simulink model "benchlink"  (R2024b)
settings: Solver=FixedStepDiscrete  StartTime=0.0  StopTime=0.005*16  RelTol=1e-3
model workspace (MAT data in the model file):
  socvcb : containers.Map (value not decoded)
values from neighbouring files (symbols this model uses):
  access = [32 0 4 36 32 0 4 36 32 0 4 36 ... (16 elements, 16x1)]    [all_variables.mat]
  qam_params =     [all_variables.mat]
undefined symbols (not defined in the file or in its folder): Add, j, QAM, rms, Shift
libraries: hdlsllib x53, simulink_need_slupdate x22, simulink x18, dspsigops x16, commdigbbndam3 x6, dsphdlmathfun2 x2, commchan3 x1, commrflib2 x1, dsphdlsigops2 x1, dspstat3 x1, dsphdlfiltering2 x1, simulink_extras x1
(part 3 of 5)

== system benchlink/HDL_64QAM/HDLRxIPCore/QAM Rx HDL/DA CFC_Avg/Moving_Average ==
  dataIn : Inport
  Trigger : TriggerPort  VariantControl=(inherit)  PortDimensions=1
  Add1 : Sum  Inputs=+-+  OutDataTypeStr=uint16
  Constant18 : Constant  Value=0.125  OutDataTypeStr=fixdt(1,16,14)  SampleTime=-1
  Delay : Delay  DelayLength=8
  Delay4 : Delay  DelayLength=1  InitialCondition=0  UseCircularBuffer=on
  Product : Product
  Time Scope : Scope  NumInputPorts=4
  to int1 : DataTypeConversion  OutDataTypeStr=int16  RndMeth=Floor
  to int2 : DataTypeConversion  Commented=through  OutDataTypeStr=int32  RndMeth=Floor
  dataOut : Outport  InitialOutput=0  VectorParamsAs1DForOutWhenUnconnected=off
  wires:
  dataIn/1 -> to int2/1
  Delay4/1 -> Add1/1
  Product/1 -> to int1/1
  to int1/1 -> Time Scope/4, dataOut/1
  Delay/1 -> Time Scope/2, Add1/2
  Add1/1 -> Time Scope/3, Product/1, Delay4/1
  to int2/1 -> Time Scope/1, Add1/3, Delay/1
  Constant18/1 -> Product/2

== system benchlink/HDL_64QAM/HDLRxIPCore/QAM Rx HDL/EB Downsampler by 6/Modulus ==
  note: sqrt(I^2+Q^2) can be approximated as |L|+0.4*|S|,
      | where |L| is the absolute value of the larger of I or Q,
      | and |S| is the absolute value of the smaller of I or Q.
      |
      | See "|L|+0.4|S| Algorithm" on page 238 in "Digital Signal
      | Processing in Communication Systems" by Marvin Frerking.
  dataIn : Inport
  Abs : Abs
  Abs1 : Abs
  Add7 : Sum  SaturateOnIntegerOverflow=on
  Complex to Real-Imag2 : ComplexToRealImag
  Delay{1..7} (7 alike) : Delay  DelayLength=1  InitialCondition=0
  Gain4 : Gain  Gain=0.4  OutDataTypeStr=fixdt(1,16,15)  SaturateOnIntegerOverflow=on
  MinMax : MinMax  Inputs=2  SaturateOnIntegerOverflow=on
  MinMax1 : MinMax  Function=max  Inputs=2  SaturateOnIntegerOverflow=on
  dataOut : Outport  VectorParamsAs1DForOutWhenUnconnected=off
  wires:
  dataIn/1 -> Complex to Real-Imag2/1
  Abs1/1 -> Delay1/1
  Abs/1 -> Delay4/1
  Gain4/1 -> Delay6/1
  MinMax1/1 -> Delay2/1  "|L|"
  MinMax/1 -> Delay7/1  "|Q|"
  Add7/1 -> Delay5/1
  Delay7/1 -> Gain4/1
  Delay2/1 -> Delay3/1
  Delay1/1 -> MinMax1/2, MinMax/2
  Delay4/1 -> MinMax1/1, MinMax/1
  Delay6/1 -> Add7/2
  Delay5/1 -> dataOut/1
  Delay3/1 -> Add7/1
  Complex to Real-Imag2/2 -> Abs1/1  "Q"
  Complex to Real-Imag2/1 -> Abs/1  "I"

== system benchlink/HDL_64QAM/HDLRxIPCore/QAM Rx HDL/EB Downsampler by 6/Moving_Average ==
  dataIn : Inport
  Add : Sum  Inputs=-+  AccumDataTypeStr=fixdt(1,32,18)
  Add1 : Sum  OutDataTypeStr=fixdt(1,32,18)  AccumDataTypeStr=fixdt(1,32,18)
  Delay : Delay  DelayLength=M-1
  Delay10 : Delay  DelayLength=1  InitialCondition=0  UseCircularBuffer=on
  Delay4 : Delay  DelayLength=1  InitialCondition=0  UseCircularBuffer=on
  Gain : Gain  OutDataTypeStr=fixdt(1,32,23)
  dataOut : Outport  VectorParamsAs1DForOutWhenUnconnected=off
  wires:
  Add/1 -> Delay10/1
  dataIn/1 -> Delay/1, Add/2
  Delay10/1 -> Add1/2
  Add1/1 -> Gain/1, Delay4/1
  Delay/1 -> Add/1
  Delay4/1 -> Add1/1
  Gain/1 -> dataOut/1

== system benchlink/HDL_64QAM/HDLRxIPCore/QAM Rx HDL/EB Downsampler by 6_Old2/Modulus ==
  note: sqrt(I^2+Q^2) can be approximated as |L|+0.4*|S|,
      | where |L| is the absolute value of the larger of I or Q,
      | and |S| is the absolute value of the smaller of I or Q.
      |
      | See "|L|+0.4|S| Algorithm" on page 238 in "Digital Signal
      | Processing in Communication Systems" by Marvin Frerking.
  dataIn : Inport
  Abs : Abs
  Abs1 : Abs
  Add7 : Sum  SaturateOnIntegerOverflow=on
  Complex to Real-Imag2 : ComplexToRealImag
  Delay{1..7} (7 alike) : Delay  DelayLength=1  InitialCondition=0
  Gain4 : Gain  Gain=0.4  OutDataTypeStr=fixdt(1,16,15)  SaturateOnIntegerOverflow=on
  MinMax : MinMax  Inputs=2  SaturateOnIntegerOverflow=on
  MinMax1 : MinMax  Function=max  Inputs=2  SaturateOnIntegerOverflow=on
  dataOut : Outport  VectorParamsAs1DForOutWhenUnconnected=off
  wires:
  dataIn/1 -> Complex to Real-Imag2/1
  Abs1/1 -> Delay1/1
  Abs/1 -> Delay4/1
  Gain4/1 -> Delay6/1
  MinMax1/1 -> Delay2/1  "|L|"
  MinMax/1 -> Delay7/1  "|Q|"
  Add7/1 -> Delay5/1
  Delay7/1 -> Gain4/1
  Delay2/1 -> Delay3/1
  Delay1/1 -> MinMax1/2, MinMax/2
  Delay4/1 -> MinMax1/1, MinMax/1
  Delay6/1 -> Add7/2
  Delay5/1 -> dataOut/1
  Delay3/1 -> Add7/1
  Complex to Real-Imag2/2 -> Abs1/1  "Q"
  Complex to Real-Imag2/1 -> Abs/1  "I"

== system benchlink/HDL_64QAM/HDLRxIPCore/QAM Rx HDL/EB Downsampler by 6_Old2/Modulus1 ==
  note: sqrt(I^2+Q^2) can be approximated as |L|+0.4*|S|,
      | where |L| is the absolute value of the larger of I or Q,
      | and |S| is the absolute value of the smaller of I or Q.
      |
      | See "|L|+0.4|S| Algorithm" on page 238 in "Digital Signal
      | Processing in Communication Systems" by Marvin Frerking.
  dataIn : Inport
  Abs : Abs
  Abs1 : Abs
  Add7 : Sum  SaturateOnIntegerOverflow=on
  Complex to Real-Imag2 : ComplexToRealImag
  Delay{1..7} (7 alike) : Delay  DelayLength=1  InitialCondition=0
  Gain4 : Gain  Gain=0.4  OutDataTypeStr=fixdt(1,16,15)  SaturateOnIntegerOverflow=on
  MinMax : MinMax  Inputs=2  SaturateOnIntegerOverflow=on
  MinMax1 : MinMax  Function=max  Inputs=2  SaturateOnIntegerOverflow=on
  dataOut : Outport  VectorParamsAs1DForOutWhenUnconnected=off
  wires:
  dataIn/1 -> Complex to Real-Imag2/1
  Abs1/1 -> Delay1/1
  Abs/1 -> Delay4/1
  Gain4/1 -> Delay6/1
  MinMax1/1 -> Delay2/1  "|L|"
  MinMax/1 -> Delay7/1  "|Q|"
  Add7/1 -> Delay5/1
  Delay7/1 -> Gain4/1
  Delay2/1 -> Delay3/1
  Delay1/1 -> MinMax1/2, MinMax/2
  Delay4/1 -> MinMax1/1, MinMax/1
  Delay6/1 -> Add7/2
  Delay5/1 -> dataOut/1
  Delay3/1 -> Add7/1
  Complex to Real-Imag2/2 -> Abs1/1  "Q"
  Complex to Real-Imag2/1 -> Abs/1  "I"

== system benchlink/HDL_64QAM/HDLRxIPCore/QAM Rx HDL/EB Downsampler by 6_Old2/Modulus2 ==
  note: sqrt(I^2+Q^2) can be approximated as |L|+0.4*|S|,
      | where |L| is the absolute value of the larger of I or Q,
      | and |S| is the absolute value of the smaller of I or Q.
      |
      | See "|L|+0.4|S| Algorithm" on page 238 in "Digital Signal
      | Processing in Communication Systems" by Marvin Frerking.
  dataIn : Inport
  Abs : Abs
  Abs1 : Abs
  Add7 : Sum  SaturateOnIntegerOverflow=on
  Complex to Real-Imag2 : ComplexToRealImag
  Delay{1..7} (7 alike) : Delay  DelayLength=1  InitialCondition=0
  Gain4 : Gain  Gain=0.4  OutDataTypeStr=fixdt(1,16,15)  SaturateOnIntegerOverflow=on
  MinMax : MinMax  Inputs=2  SaturateOnIntegerOverflow=on
  MinMax1 : MinMax  Function=max  Inputs=2  SaturateOnIntegerOverflow=on
  dataOut : Outport  VectorParamsAs1DForOutWhenUnconnected=off
  wires:
  dataIn/1 -> Complex to Real-Imag2/1
  Abs1/1 -> Delay1/1
  Abs/1 -> Delay4/1
  Gain4/1 -> Delay6/1
  MinMax1/1 -> Delay2/1  "|L|"
  MinMax/1 -> Delay7/1  "|Q|"
  Add7/1 -> Delay5/1
  Delay7/1 -> Gain4/1
  Delay2/1 -> Delay3/1
  Delay1/1 -> MinMax1/2, MinMax/2
  Delay4/1 -> MinMax1/1, MinMax/1
  Delay6/1 -> Add7/2
  Delay5/1 -> dataOut/1
  Delay3/1 -> Add7/1
  Complex to Real-Imag2/2 -> Abs1/1  "Q"
  Complex to Real-Imag2/1 -> Abs/1  "I"

== system benchlink/HDL_64QAM/HDLRxIPCore/QAM Rx HDL/EB Downsampler by 6_Old2/Modulus3 ==
  note: sqrt(I^2+Q^2) can be approximated as |L|+0.4*|S|,
      | where |L| is the absolute value of the larger of I or Q,
      | and |S| is the absolute value of the smaller of I or Q.
      |
      | See "|L|+0.4|S| Algorithm" on page 238 in "Digital Signal
      | Processing in Communication Systems" by Marvin Frerking.
  dataIn : Inport
  Abs : Abs
  Abs1 : Abs
  Add7 : Sum  SaturateOnIntegerOverflow=on
  Complex to Real-Imag2 : ComplexToRealImag
  Delay{1..7} (7 alike) : Delay  DelayLength=1  InitialCondition=0
  Gain4 : Gain  Gain=0.4  OutDataTypeStr=fixdt(1,16,15)  SaturateOnIntegerOverflow=on
  MinMax : MinMax  Inputs=2  SaturateOnIntegerOverflow=on
  MinMax1 : MinMax  Function=max  Inputs=2  SaturateOnIntegerOverflow=on
  dataOut : Outport  VectorParamsAs1DForOutWhenUnconnected=off
  wires:
  dataIn/1 -> Complex to Real-Imag2/1
  Abs1/1 -> Delay1/1
  Abs/1 -> Delay4/1
  Gain4/1 -> Delay6/1
  MinMax1/1 -> Delay2/1  "|L|"
  MinMax/1 -> Delay7/1  "|Q|"
  Add7/1 -> Delay5/1
  Delay7/1 -> Gain4/1
  Delay2/1 -> Delay3/1
  Delay1/1 -> MinMax1/2, MinMax/2
  Delay4/1 -> MinMax1/1, MinMax/1
  Delay6/1 -> Add7/2
  Delay5/1 -> dataOut/1
  Delay3/1 -> Add7/1
  Complex to Real-Imag2/2 -> Abs1/1  "Q"
  Complex to Real-Imag2/1 -> Abs/1  "I"

== system benchlink/HDL_64QAM/HDLRxIPCore/QAM Rx HDL/EB Downsampler by 6_Old2/Modulus4 ==
  note: sqrt(I^2+Q^2) can be approximated as |L|+0.4*|S|,
      | where |L| is the absolute value of the larger of I or Q,
      | and |S| is the absolute value of the smaller of I or Q.
      |
      | See "|L|+0.4|S| Algorithm" on page 238 in "Digital Signal
      | Processing in Communication Systems" by Marvin Frerking.
  dataIn : Inport
  Abs : Abs
  Abs1 : Abs
  Add7 : Sum  SaturateOnIntegerOverflow=on
  Complex to Real-Imag2 : ComplexToRealImag
  Delay{1..7} (7 alike) : Delay  DelayLength=1  InitialCondition=0
  Gain4 : Gain  Gain=0.4  OutDataTypeStr=fixdt(1,16,15)  SaturateOnIntegerOverflow=on
  MinMax : MinMax  Inputs=2  SaturateOnIntegerOverflow=on
  MinMax1 : MinMax  Function=max  Inputs=2  SaturateOnIntegerOverflow=on
  dataOut : Outport  VectorParamsAs1DForOutWhenUnconnected=off
  wires:
  dataIn/1 -> Complex to Real-Imag2/1
  Abs1/1 -> Delay1/1
  Abs/1 -> Delay4/1
  Gain4/1 -> Delay6/1
  MinMax1/1 -> Delay2/1  "|L|"
  MinMax/1 -> Delay7/1  "|Q|"
  Add7/1 -> Delay5/1
  Delay7/1 -> Gain4/1
  Delay2/1 -> Delay3/1
  Delay1/1 -> MinMax1/2, MinMax/2
  Delay4/1 -> MinMax1/1, MinMax/1
  Delay6/1 -> Add7/2
  Delay5/1 -> dataOut/1
  Delay3/1 -> Add7/1
  Complex to Real-Imag2/2 -> Abs1/1  "Q"
  Complex to Real-Imag2/1 -> Abs/1  "I"

== system benchlink/HDL_64QAM/HDLRxIPCore/QAM Rx HDL/EB Downsampler by 6_Old2/Modulus5 ==
  note: sqrt(I^2+Q^2) can be approximated as |L|+0.4*|S|,
      | where |L| is the absolute value of the larger of I or Q,
      | and |S| is the absolute value of the smaller of I or Q.
      |
      | See "|L|+0.4|S| Algorithm" on page 238 in "Digital Signal
      | Processing in Communication Systems" by Marvin Frerking.
  dataIn : Inport
  Abs : Abs
  Abs1 : Abs
  Add7 : Sum  SaturateOnIntegerOverflow=on
  Complex to Real-Imag2 : ComplexToRealImag
  Delay{1..7} (7 alike) : Delay  DelayLength=1  InitialCondition=0
  Gain4 : Gain  Gain=0.4  OutDataTypeStr=fixdt(1,16,15)  SaturateOnIntegerOverflow=on
  MinMax : MinMax  Inputs=2  SaturateOnIntegerOverflow=on
  MinMax1 : MinMax  Function=max  Inputs=2  SaturateOnIntegerOverflow=on
  dataOut : Outport  VectorParamsAs1DForOutWhenUnconnected=off
  wires:
  dataIn/1 -> Complex to Real-Imag2/1
  Abs1/1 -> Delay1/1
  Abs/1 -> Delay4/1
  Gain4/1 -> Delay6/1
  MinMax1/1 -> Delay2/1  "|L|"
  MinMax/1 -> Delay7/1  "|Q|"
  Add7/1 -> Delay5/1
  Delay7/1 -> Gain4/1
  Delay2/1 -> Delay3/1
  Delay1/1 -> MinMax1/2, MinMax/2
  Delay4/1 -> MinMax1/1, MinMax/1
  Delay6/1 -> Add7/2
  Delay5/1 -> dataOut/1
  Delay3/1 -> Add7/1
  Complex to Real-Imag2/2 -> Abs1/1  "Q"
  Complex to Real-Imag2/1 -> Abs/1  "I"

== system benchlink/HDL_64QAM/HDLRxIPCore/QAM Rx HDL/EB Downsampler by 6_Old2/Moving_Average ==
  dataIn : Inport
  Add : Sum  Inputs=-+  AccumDataTypeStr=fixdt(1,32,18)
  Add1 : Sum  OutDataTypeStr=fixdt(1,32,18)  AccumDataTypeStr=fixdt(1,32,18)
  Delay : Delay  DelayLength=M-1
  Delay10 : Delay  DelayLength=1  InitialCondition=0  UseCircularBuffer=on
  Delay4 : Delay  DelayLength=1  InitialCondition=0  UseCircularBuffer=on
  Gain : Gain  OutDataTypeStr=fixdt(1,32,23)
  dataOut : Outport  VectorParamsAs1DForOutWhenUnconnected=off
  wires:
  Add/1 -> Delay10/1
  dataIn/1 -> Delay/1, Add/2
  Delay10/1 -> Add1/2
  Add1/1 -> Gain/1, Delay4/1
  Delay/1 -> Add/1
  Delay4/1 -> Add1/1
  Gain/1 -> dataOut/1

== system benchlink/HDL_64QAM/HDLRxIPCore/QAM Rx HDL/EB Downsampler by 6_Old2/Moving_Average1 ==
  dataIn : Inport
  Add : Sum  Inputs=-+  AccumDataTypeStr=fixdt(1,32,18)
  Add1 : Sum  OutDataTypeStr=fixdt(1,32,18)  AccumDataTypeStr=fixdt(1,32,18)
  Delay : Delay  DelayLength=M-1
  Delay10 : Delay  DelayLength=1  InitialCondition=0  UseCircularBuffer=on
  Delay4 : Delay  DelayLength=1  InitialCondition=0  UseCircularBuffer=on
  Gain : Gain  OutDataTypeStr=fixdt(1,32,23)
  dataOut : Outport  VectorParamsAs1DForOutWhenUnconnected=off
  wires:
  Add/1 -> Delay10/1
  dataIn/1 -> Delay/1, Add/2
  Delay10/1 -> Add1/2
  Add1/1 -> Gain/1, Delay4/1
  Delay/1 -> Add/1
  Delay4/1 -> Add1/1
  Gain/1 -> dataOut/1

== system benchlink/HDL_64QAM/HDLRxIPCore/QAM Rx HDL/EB Downsampler by 6_Old2/Moving_Average2 ==
  dataIn : Inport
  Add : Sum  Inputs=-+  AccumDataTypeStr=fixdt(1,32,18)
  Add1 : Sum  OutDataTypeStr=fixdt(1,32,18)  AccumDataTypeStr=fixdt(1,32,18)
  Delay : Delay  DelayLength=M-1
  Delay10 : Delay  DelayLength=1  InitialCondition=0  UseCircularBuffer=on
  Delay4 : Delay  DelayLength=1  InitialCondition=0  UseCircularBuffer=on
  Gain : Gain  OutDataTypeStr=fixdt(1,32,23)
  dataOut : Outport  VectorParamsAs1DForOutWhenUnconnected=off
  wires:
  Add/1 -> Delay10/1
  dataIn/1 -> Delay/1, Add/2
  Delay10/1 -> Add1/2
  Add1/1 -> Gain/1, Delay4/1
  Delay/1 -> Add/1
  Delay4/1 -> Add1/1
  Gain/1 -> dataOut/1

== system benchlink/HDL_64QAM/HDLRxIPCore/QAM Rx HDL/EB Downsampler by 6_Old2/Moving_Average3 ==
  dataIn : Inport
  Add : Sum  Inputs=-+  AccumDataTypeStr=fixdt(1,32,18)
  Add1 : Sum  OutDataTypeStr=fixdt(1,32,18)  AccumDataTypeStr=fixdt(1,32,18)
  Delay : Delay  DelayLength=M-1
  Delay10 : Delay  DelayLength=1  InitialCondition=0  UseCircularBuffer=on
  Delay4 : Delay  DelayLength=1  InitialCondition=0  UseCircularBuffer=on
  Gain : Gain  OutDataTypeStr=fixdt(1,32,23)
  dataOut : Outport  VectorParamsAs1DForOutWhenUnconnected=off
  wires:
  Add/1 -> Delay10/1
  dataIn/1 -> Delay/1, Add/2
  Delay10/1 -> Add1/2
  Add1/1 -> Gain/1, Delay4/1
  Delay/1 -> Add/1
  Delay4/1 -> Add1/1
  Gain/1 -> dataOut/1

== system benchlink/HDL_64QAM/HDLRxIPCore/QAM Rx HDL/EB Downsampler by 6_Old2/Moving_Average4 ==
  dataIn : Inport
  Add : Sum  Inputs=-+  AccumDataTypeStr=fixdt(1,32,18)
  Add1 : Sum  OutDataTypeStr=fixdt(1,32,18)  AccumDataTypeStr=fixdt(1,32,18)
  Delay : Delay  DelayLength=M-1
  Delay10 : Delay  DelayLength=1  InitialCondition=0  UseCircularBuffer=on
  Delay4 : Delay  DelayLength=1  InitialCondition=0  UseCircularBuffer=on
  Gain : Gain  OutDataTypeStr=fixdt(1,32,23)
  dataOut : Outport  VectorParamsAs1DForOutWhenUnconnected=off
  wires:
  Add/1 -> Delay10/1
  dataIn/1 -> Delay/1, Add/2
  Delay10/1 -> Add1/2
  Add1/1 -> Gain/1, Delay4/1
  Delay/1 -> Add/1
  Delay4/1 -> Add1/1
  Gain/1 -> dataOut/1

== system benchlink/HDL_64QAM/HDLRxIPCore/QAM Rx HDL/EB Downsampler by 6_Old2/Moving_Average5 ==
  dataIn : Inport
  Add : Sum  Inputs=-+  AccumDataTypeStr=fixdt(1,32,18)
  Add1 : Sum  OutDataTypeStr=fixdt(1,32,18)  AccumDataTypeStr=fixdt(1,32,18)
  Delay : Delay  DelayLength=M-1
  Delay10 : Delay  DelayLength=1  InitialCondition=0  UseCircularBuffer=on
  Delay4 : Delay  DelayLength=1  InitialCondition=0  UseCircularBuffer=on
  Gain : Gain  OutDataTypeStr=fixdt(1,32,23)
  dataOut : Outport  VectorParamsAs1DForOutWhenUnconnected=off
  wires:
  Add/1 -> Delay10/1
  dataIn/1 -> Delay/1, Add/2
  Delay10/1 -> Add1/2
  Add1/1 -> Gain/1, Delay4/1
  Delay/1 -> Add/1
  Delay4/1 -> Add1/1
  Gain/1 -> dataOut/1

== system benchlink/HDL_64QAM/HDLRxIPCore/QAM Rx HDL/EB Downsampler by 6_old/Modulus ==
  note: sqrt(I^2+Q^2) can be approximated as |L|+0.4*|S|,
      | where |L| is the absolute value of the larger of I or Q,
      | and |S| is the absolute value of the smaller of I or Q.
      |
      | See "|L|+0.4|S| Algorithm" on page 238 in "Digital Signal
      | Processing in Communication Systems" by Marvin Frerking.
  dataIn : Inport
  Abs : Abs
  Abs1 : Abs
  Add7 : Sum  SaturateOnIntegerOverflow=on
  Complex to Real-Imag2 : ComplexToRealImag
  Delay{1..7} (7 alike) : Delay  DelayLength=1  InitialCondition=0
  Gain4 : Gain  Gain=0.4  OutDataTypeStr=fixdt(1,16,15)  SaturateOnIntegerOverflow=on
  MinMax : MinMax  Inputs=2  SaturateOnIntegerOverflow=on
  MinMax1 : MinMax  Function=max  Inputs=2  SaturateOnIntegerOverflow=on
  dataOut : Outport  VectorParamsAs1DForOutWhenUnconnected=off
  wires:
  dataIn/1 -> Complex to Real-Imag2/1
  Abs1/1 -> Delay1/1
  Abs/1 -> Delay4/1
  Gain4/1 -> Delay6/1
  MinMax1/1 -> Delay2/1  "|L|"
  MinMax/1 -> Delay7/1  "|Q|"
  Add7/1 -> Delay5/1
  Delay7/1 -> Gain4/1
  Delay2/1 -> Delay3/1
  Delay1/1 -> MinMax1/2, MinMax/2
  Delay4/1 -> MinMax1/1, MinMax/1
  Delay6/1 -> Add7/2
  Delay5/1 -> dataOut/1
  Delay3/1 -> Add7/1
  Complex to Real-Imag2/2 -> Abs1/1  "Q"
  Complex to Real-Imag2/1 -> Abs/1  "I"

== system benchlink/HDL_64QAM/HDLRxIPCore/QAM Rx HDL/EB Downsampler by 6_old/Modulus1 ==
  note: sqrt(I^2+Q^2) can be approximated as |L|+0.4*|S|,
      | where |L| is the absolute value of the larger of I or Q,
      | and |S| is the absolute value of the smaller of I or Q.
      |
      | See "|L|+0.4|S| Algorithm" on page 238 in "Digital Signal
      | Processing in Communication Systems" by Marvin Frerking.
  dataIn : Inport
  Abs : Abs
  Abs1 : Abs
  Add7 : Sum  SaturateOnIntegerOverflow=on
  Complex to Real-Imag2 : ComplexToRealImag
  Delay{1..7} (7 alike) : Delay  DelayLength=1  InitialCondition=0
  Gain4 : Gain  Gain=0.4  OutDataTypeStr=fixdt(1,16,15)  SaturateOnIntegerOverflow=on
  MinMax : MinMax  Inputs=2  SaturateOnIntegerOverflow=on
  MinMax1 : MinMax  Function=max  Inputs=2  SaturateOnIntegerOverflow=on
  dataOut : Outport  VectorParamsAs1DForOutWhenUnconnected=off
  wires:
  dataIn/1 -> Complex to Real-Imag2/1
  Abs1/1 -> Delay1/1
  Abs/1 -> Delay4/1
  Gain4/1 -> Delay6/1
  MinMax1/1 -> Delay2/1  "|L|"
  MinMax/1 -> Delay7/1  "|Q|"
  Add7/1 -> Delay5/1
  Delay7/1 -> Gain4/1
  Delay2/1 -> Delay3/1
  Delay1/1 -> MinMax1/2, MinMax/2
  Delay4/1 -> MinMax1/1, MinMax/1
  Delay6/1 -> Add7/2
  Delay5/1 -> dataOut/1
  Delay3/1 -> Add7/1
  Complex to Real-Imag2/2 -> Abs1/1  "Q"
  Complex to Real-Imag2/1 -> Abs/1  "I"

== system benchlink/HDL_64QAM/HDLRxIPCore/QAM Rx HDL/EB Downsampler by 6_old/Modulus2 ==
  note: sqrt(I^2+Q^2) can be approximated as |L|+0.4*|S|,
      | where |L| is the absolute value of the larger of I or Q,
      | and |S| is the absolute value of the smaller of I or Q.
      |
      | See "|L|+0.4|S| Algorithm" on page 238 in "Digital Signal
      | Processing in Communication Systems" by Marvin Frerking.
  dataIn : Inport
  Abs : Abs
  Abs1 : Abs
  Add7 : Sum  SaturateOnIntegerOverflow=on
  Complex to Real-Imag2 : ComplexToRealImag
  Delay{1..7} (7 alike) : Delay  DelayLength=1  InitialCondition=0
  Gain4 : Gain  Gain=0.4  OutDataTypeStr=fixdt(1,16,15)  SaturateOnIntegerOverflow=on
  MinMax : MinMax  Inputs=2  SaturateOnIntegerOverflow=on
  MinMax1 : MinMax  Function=max  Inputs=2  SaturateOnIntegerOverflow=on
  dataOut : Outport  VectorParamsAs1DForOutWhenUnconnected=off
  wires:
  dataIn/1 -> Complex to Real-Imag2/1
  Abs1/1 -> Delay1/1
  Abs/1 -> Delay4/1
  Gain4/1 -> Delay6/1
  MinMax1/1 -> Delay2/1  "|L|"
  MinMax/1 -> Delay7/1  "|Q|"
  Add7/1 -> Delay5/1
  Delay7/1 -> Gain4/1
  Delay2/1 -> Delay3/1
  Delay1/1 -> MinMax1/2, MinMax/2
  Delay4/1 -> MinMax1/1, MinMax/1
  Delay6/1 -> Add7/2
  Delay5/1 -> dataOut/1
  Delay3/1 -> Add7/1
  Complex to Real-Imag2/2 -> Abs1/1  "Q"
  Complex to Real-Imag2/1 -> Abs/1  "I"

== system benchlink/HDL_64QAM/HDLRxIPCore/QAM Rx HDL/EB Downsampler by 6_old/Modulus3 ==
  note: sqrt(I^2+Q^2) can be approximated as |L|+0.4*|S|,
      | where |L| is the absolute value of the larger of I or Q,
      | and |S| is the absolute value of the smaller of I or Q.
      |
      | See "|L|+0.4|S| Algorithm" on page 238 in "Digital Signal
      | Processing in Communication Systems" by Marvin Frerking.
  dataIn : Inport
  Abs : Abs
  Abs1 : Abs
  Add7 : Sum  SaturateOnIntegerOverflow=on
  Complex to Real-Imag2 : ComplexToRealImag
  Delay{1..7} (7 alike) : Delay  DelayLength=1  InitialCondition=0
  Gain4 : Gain  Gain=0.4  OutDataTypeStr=fixdt(1,16,15)  SaturateOnIntegerOverflow=on
  MinMax : MinMax  Inputs=2  SaturateOnIntegerOverflow=on
  MinMax1 : MinMax  Function=max  Inputs=2  SaturateOnIntegerOverflow=on
  dataOut : Outport  VectorParamsAs1DForOutWhenUnconnected=off
  wires:
  dataIn/1 -> Complex to Real-Imag2/1
  Abs1/1 -> Delay1/1
  Abs/1 -> Delay4/1
  Gain4/1 -> Delay6/1
  MinMax1/1 -> Delay2/1  "|L|"
  MinMax/1 -> Delay7/1  "|Q|"
  Add7/1 -> Delay5/1
  Delay7/1 -> Gain4/1
  Delay2/1 -> Delay3/1
  Delay1/1 -> MinMax1/2, MinMax/2
  Delay4/1 -> MinMax1/1, MinMax/1
  Delay6/1 -> Add7/2
  Delay5/1 -> dataOut/1
  Delay3/1 -> Add7/1
  Complex to Real-Imag2/2 -> Abs1/1  "Q"
  Complex to Real-Imag2/1 -> Abs/1  "I"

== system benchlink/HDL_64QAM/HDLRxIPCore/QAM Rx HDL/EB Downsampler by 6_old/Modulus4 ==
  note: sqrt(I^2+Q^2) can be approximated as |L|+0.4*|S|,
      | where |L| is the absolute value of the larger of I or Q,
      | and |S| is the absolute value of the smaller of I or Q.
      |
      | See "|L|+0.4|S| Algorithm" on page 238 in "Digital Signal
      | Processing in Communication Systems" by Marvin Frerking.
  dataIn : Inport
  Abs : Abs
  Abs1 : Abs
  Add7 : Sum  SaturateOnIntegerOverflow=on
  Complex to Real-Imag2 : ComplexToRealImag
  Delay{1..7} (7 alike) : Delay  DelayLength=1  InitialCondition=0
  Gain4 : Gain  Gain=0.4  OutDataTypeStr=fixdt(1,16,15)  SaturateOnIntegerOverflow=on
  MinMax : MinMax  Inputs=2  SaturateOnIntegerOverflow=on
  MinMax1 : MinMax  Function=max  Inputs=2  SaturateOnIntegerOverflow=on
  dataOut : Outport  VectorParamsAs1DForOutWhenUnconnected=off
  wires:
  dataIn/1 -> Complex to Real-Imag2/1
  Abs1/1 -> Delay1/1
  Abs/1 -> Delay4/1
  Gain4/1 -> Delay6/1
  MinMax1/1 -> Delay2/1  "|L|"
  MinMax/1 -> Delay7/1  "|Q|"
  Add7/1 -> Delay5/1
  Delay7/1 -> Gain4/1
  Delay2/1 -> Delay3/1
  Delay1/1 -> MinMax1/2, MinMax/2
  Delay4/1 -> MinMax1/1, MinMax/1
  Delay6/1 -> Add7/2
  Delay5/1 -> dataOut/1
  Delay3/1 -> Add7/1
  Complex to Real-Imag2/2 -> Abs1/1  "Q"
  Complex to Real-Imag2/1 -> Abs/1  "I"

== system benchlink/HDL_64QAM/HDLRxIPCore/QAM Rx HDL/EB Downsampler by 6_old/Modulus5 ==
  note: sqrt(I^2+Q^2) can be approximated as |L|+0.4*|S|,
      | where |L| is the absolute value of the larger of I or Q,
      | and |S| is the absolute value of the smaller of I or Q.
      |
      | See "|L|+0.4|S| Algorithm" on page 238 in "Digital Signal
      | Processing in Communication Systems" by Marvin Frerking.
  dataIn : Inport
  Abs : Abs
  Abs1 : Abs
  Add7 : Sum  SaturateOnIntegerOverflow=on
  Complex to Real-Imag2 : ComplexToRealImag
  Delay{1..7} (7 alike) : Delay  DelayLength=1  InitialCondition=0
  Gain4 : Gain  Gain=0.4  OutDataTypeStr=fixdt(1,16,15)  SaturateOnIntegerOverflow=on
  MinMax : MinMax  Inputs=2  SaturateOnIntegerOverflow=on
  MinMax1 : MinMax  Function=max  Inputs=2  SaturateOnIntegerOverflow=on
  dataOut : Outport  VectorParamsAs1DForOutWhenUnconnected=off
  wires:
  dataIn/1 -> Complex to Real-Imag2/1
  Abs1/1 -> Delay1/1
  Abs/1 -> Delay4/1
  Gain4/1 -> Delay6/1
  MinMax1/1 -> Delay2/1  "|L|"
  MinMax/1 -> Delay7/1  "|Q|"
  Add7/1 -> Delay5/1
  Delay7/1 -> Gain4/1
  Delay2/1 -> Delay3/1
  Delay1/1 -> MinMax1/2, MinMax/2
  Delay4/1 -> MinMax1/1, MinMax/1
  Delay6/1 -> Add7/2
  Delay5/1 -> dataOut/1
  Delay3/1 -> Add7/1
  Complex to Real-Imag2/2 -> Abs1/1  "Q"
  Complex to Real-Imag2/1 -> Abs/1  "I"

== system benchlink/HDL_64QAM/HDLRxIPCore/QAM Rx HDL/Enabled AGC1/Energy Detector ==
  In : Inport
  Add1 : Sum  Inputs=+-  OutDataTypeStr=fixdt(1,64,46)  AccumDataTypeStr=fixdt(1,64,46)
  Bit Shift1 : hdlsllib/Logic and Bit Operations/Bit Shift  mode=Shift Right Arithmetic  N=3
  Compare To Zero1 : simulink/Logic and Bit Operations/Compare To Zero  relop=>  OutDataTypeStr=boolean
  Delay2 : Delay  DelayLength=1  InitialCondition=0  UseCircularBuffer=on
  Delay24 : Delay  DelayLength=qam_params.golayLength*qam_params.Upsampling  InitialCondition=0  UseCircularBuffer=on
  Delay3 : Delay  DelayLength=1  InitialCondition=0  UseCircularBuffer=on
  Delay5 : Delay  DelayLength=qam_params.golayLength*qam_params.Upsampling  InitialCondition=0  UseCircularBuffer=on
  Delay7 : Delay  DelayLength=1  InitialCondition=0  UseCircularBuffer=on
  Latch1 : Subsystem
  To Workspace1 : ToWorkspace  VariableName=yout473  SampleTime=-1
      settings: Save2DSignal=2-D array (concatenate along first dimension)
  To Workspace11 : ToWorkspace  VariableName=yout474  SampleTime=-1
      settings: Save2DSignal=2-D array (concatenate along first dimension)
  To Workspace15 : ToWorkspace  VariableName=yout475  SampleTime=-1
      settings: Save2DSignal=2-D array (concatenate along first dimension)
  To Workspace19 : ToWorkspace  VariableName=yout476  SampleTime=-1
      settings: Save2DSignal=2-D array (concatenate along first dimension)
  To Workspace2 : ToWorkspace  VariableName=yout477  SampleTime=-1
      settings: Save2DSignal=2-D array (concatenate along first dimension)
  Variance Estimate : Subsystem
  Variance Estimate2 : Subsystem
  Out : Outport  VectorParamsAs1DForOutWhenUnconnected=off
  wires:
  Delay5/1 -> Variance Estimate2/1(dataIn)
  Delay7/1 -> Compare To Zero1/1
  Bit Shift1/1 -> Add1/1
  Variance Estimate2/2(varAbs) -> To Workspace15/1, Delay2/1
  Latch1/1(Q) -> To Workspace19/1, Out/1
  Delay3/1 -> Bit Shift1/1
  Compare To Zero1/1 -> Delay24/1, To Workspace1/1, Latch1/1(S)
  Delay24/1 -> To Workspace2/1, Latch1/2(R)
  Add1/1 -> Delay7/1
  Variance Estimate/2(varAbs) -> To Workspace11/1, Delay3/1
  Delay2/1 -> Add1/2
  In/1 -> Delay5/1, Variance Estimate/1(dataIn)

== system benchlink/HDL_64QAM/HDLRxIPCore/QAM Rx HDL/Enabled AGC1/power ==
  In1 : Inport
  Complex to Real-Imag : ComplexToRealImag
  Delay : Delay  InitialCondition=0
  Delay1 : Delay  InitialCondition=0
  Delay3 : Delay  InitialCondition=0
  Product3 : Product  OutDataTypeStr=fixdt(1,16,15)  SaturateOnIntegerOverflow=on
  Product4 : Product  OutDataTypeStr=fixdt(1,16,15)  SaturateOnIntegerOverflow=on
  Sum1 : Sum  OutDataTypeStr=fixdt(1,16,14)  AccumDataTypeStr=fixdt(1,16,15)  SaturateOnIntegerOverflow=on
  Out1 : Outport  VectorParamsAs1DForOutWhenUnconnected=off
  wires:
  Product3/1 -> Delay/1
  Complex to Real-Imag/1 -> Product3/2, Product3/1
  Complex to Real-Imag/2 -> Product4/1, Product4/2
  Product4/1 -> Delay1/1
  Sum1/1 -> Delay3/1
  Delay/1 -> Sum1/1
  Delay1/1 -> Sum1/2
  In1/1 -> Complex to Real-Imag/1
  Delay3/1 -> Out1/1

== system benchlink/HDL_64QAM/HDLRxIPCore/QAM Rx HDL/Enabled AGC2/Energy Detector ==
  In : Inport
  Add1 : Sum  Inputs=+-  OutDataTypeStr=fixdt(1,64,46)  AccumDataTypeStr=fixdt(1,64,46)
  Add2 : Sum  Inputs=+-  OutDataTypeStr=fixdt(1,64,46)  AccumDataTypeStr=fixdt(1,64,46)
  Bit Shift1 : hdlsllib/Logic and Bit Operations/Bit Shift  mode=Shift Right Arithmetic  N=3
  Bit Shift2 : hdlsllib/Logic and Bit Operations/Bit Shift  mode=Shift Right Arithmetic  N=3
  Compare To Zero1 : simulink/Logic and Bit Operations/Compare To Zero  relop=>  OutDataTypeStr=boolean
  Compare To Zero2 : simulink/Logic and Bit Operations/Compare To Zero  relop=<  OutDataTypeStr=boolean
  Delay{1..3,7} (4 alike) : Delay  DelayLength=1  InitialCondition=0  UseCircularBuffer=on
  Delay5 : Delay  DelayLength=qam_params.golayLength*qam_params.Upsampling  InitialCondition=0  UseCircularBuffer=on
  Latch1 : Subsystem
  Variance Estimate : Subsystem
  Variance Estimate2 : Subsystem
  trigger : Outport  VectorParamsAs1DForOutWhenUnconnected=off
  wires:
  Delay5/1 -> Variance Estimate2/1(dataIn)
  Delay7/1 -> Compare To Zero1/1
  Bit Shift1/1 -> Add1/1
  Variance Estimate2/2(varAbs) -> Delay2/1
  Latch1/1(Q) -> trigger/1
  Delay3/1 -> Add2/1, Bit Shift1/1
  Compare To Zero1/1 -> Latch1/1(S)
  Compare To Zero2/1 -> Latch1/2(R)
  Add1/1 -> Delay7/1
  Variance Estimate/2(varAbs) -> Delay3/1
  Delay2/1 -> Bit Shift2/1, Add1/2
  In/1 -> Delay5/1, Variance Estimate/1(dataIn)
  Add2/1 -> Delay1/1
  Delay1/1 -> Compare To Zero2/1
  Bit Shift2/1 -> Add2/2

== system benchlink/HDL_64QAM/HDLRxIPCore/QAM Rx HDL/Enabled AGC2/power ==
  In1 : Inport
  Complex to Real-Imag : ComplexToRealImag
  Delay : Delay  InitialCondition=0
  Delay1 : Delay  InitialCondition=0
  Delay3 : Delay  InitialCondition=0
  Product3 : Product  OutDataTypeStr=fixdt(1,16,15)  SaturateOnIntegerOverflow=on
  Product4 : Product  OutDataTypeStr=fixdt(1,16,15)  SaturateOnIntegerOverflow=on
  Sum1 : Sum  OutDataTypeStr=fixdt(1,16,14)  AccumDataTypeStr=fixdt(1,16,15)  SaturateOnIntegerOverflow=on
  Out1 : Outport  VectorParamsAs1DForOutWhenUnconnected=off
  wires:
  Product3/1 -> Delay/1
  Complex to Real-Imag/1 -> Product3/2, Product3/1
  Complex to Real-Imag/2 -> Product4/1, Product4/2
  Product4/1 -> Delay1/1
  Sum1/1 -> Delay3/1
  Delay/1 -> Sum1/1
  Delay1/1 -> Sum1/2
  In1/1 -> Complex to Real-Imag/1
  Delay3/1 -> Out1/1

== system benchlink/HDL_64QAM/HDLRxIPCore/QAM Rx HDL/Enabled AGC2/signal power1 ==
  x : Inport
  trigger : Inport  Port=2
  Constant1 : Constant  Value=0  OutDataTypeStr=Inherit: Inherit via back propagation  SampleTime=1/(qam_params.sampleRate)
  Data Type Conversion : DataTypeConversion  OutDataTypeStr=fixdt(1,32,8)  SaturateOnIntegerOverflow=off  RndMeth=Floor
  Data Type Conversion1 : DataTypeConversion  OutDataTypeStr=uint32  SaturateOnIntegerOverflow=off  RndMeth=Floor
  Delay7 : Delay  DelayLength=1  InitialCondition=0  UseCircularBuffer=on  SampleTime=1/(qam_params.sampleRate)
  Logical Operator : Logic  Operator=NOT  AllPortsSameDT=off  OutDataTypeStr=boolean
  Rising Edge Detector : Subsystem
  Sum2 : Sum  Inputs=|++  OutDataTypeStr=Inherit: Same as accumulator
  Switch1 : Switch  Criteria=u2 ~= 0  SaturateOnIntegerOverflow=off  InputSameDT=off  OutDataTypeStr=Inherit: Same as first input
  Unit Delay Enabled1 : simulink_need_slupdate/Unit Delay Enabled  vinit=1  tsamp=-1
  power1 : Subsystem
  signal_power : Outport  VectorParamsAs1DForOutWhenUnconnected=off
  wires:
  Switch1/1 -> Delay7/1
  Constant1/1 -> Switch1/3
  Sum2/1 -> Switch1/1
  Rising Edge Detector/1(Out1) -> Unit Delay Enabled1/2
  Data Type Conversion/1 -> Sum2/1
  power1/1(Out1) -> Data Type Conversion/1  "magnew"
  Logical Operator/1 -> Rising Edge Detector/1(In1)
  x/1 -> power1/1(x)
  trigger/1 -> Logical Operator/1, Switch1/2
  Delay7/1 -> Unit Delay Enabled1/1, Sum2/2
  Unit Delay Enabled1/1 -> Data Type Conversion1/1
  Data Type Conversion1/1 -> signal_power/1

== system benchlink/HDL_64QAM/HDLRxIPCore/QAM Rx HDL/MF Filtering and Despreading/BER ==
  pilotValid : Inport
  pilotChips : Inport  Port=2
  chipValid : Inport  Port=3
  chips : Inport  Port=4
  Code : Inport  Port=5
  " Integrate and Dump" : MATLAB Function  TreatAsAtomicUnit=on
  " Integrate and Dump1" : MATLAB Function  TreatAsAtomicUnit=on
  BER Avg : Subsystem
  Bitwise Operator : simulink/Logic and Bit Operations/Bitwise Operator  logicop=XOR  UseBitMask=off  NumInputPorts=2  BitMask=bin2dec('11011001')  BitMaskRealWorld=Stored Integer
  Conjugate : Math  Operator=conj  SignedPower=on  RndMeth=Zero
  Data Type Conversion2 : DataTypeConversion  OutDataTypeStr=fixdt(1,16,14)  RndMeth=Floor
  Data Type Conversion3 : DataTypeConversion  OutDataTypeStr=fixdt(1,16,14)  RndMeth=Floor
  Delay10 : Delay  DelayLength=157  InitialCondition=0  UseCircularBuffer=on
  Delay{6,11,13..14,16..22} (11 alike) : Delay  DelayLength=1  InitialCondition=0  UseCircularBuffer=on
  Delay12 : Delay  DelayLength=4  InitialCondition=0  UseCircularBuffer=on
  Delay15 : Delay  DelayLength=5  InitialCondition=0  UseCircularBuffer=on
  Delay9 : Delay  DelayLength=156  InitialCondition=0  UseCircularBuffer=on
  Product2 : Product  OutDataTypeStr=fixdt(1,16,15)  RndMeth=Zero
  Rectangular QAM Demodulator Baseband1 : commdigbbndam3/Rectangular QAM Demodulator Baseband  M=64  OutType=Bit  DecType=Hard decision  VarSource=Dialog  Variance=1  Dec=Gray  Mapping=[0:15]  PowType=Min. distance between symbols  MinDist=2  AvgPow=0.66  PeakPow=1  Ph=0  outDtype1=boolean  outDtype2=Inherit via internal rule  derotateFactorWordLen=16  derotateFactorDataTypeStr=Inherit: Same word length as input  derotateFactorLastDataTypeStr=Inherit: Same word length as input  denormFactorWordLen=16  denormFactorDataTypeStr=Inherit: Same word length as input  denormFactorLastDataTypeStr=Inherit: Same word length as input  prodOutWordLen=32  prodOutOverflowMode=Wrap  prodOutRoundingMode=Floor  prodOutOvFlMode=off  prodOutOvFlModeLastStrValue=off  sumWordLen=32
  Rectangular QAM Demodulator Baseband2 : commdigbbndam3/Rectangular QAM Demodulator Baseband  M=64  OutType=Bit  DecType=Hard decision  VarSource=Dialog  Variance=1  Dec=Gray  Mapping=[0:15]  PowType=Min. distance between symbols  MinDist=2  AvgPow=0.66  PeakPow=1  Ph=0  outDtype1=boolean  outDtype2=Inherit via internal rule  derotateFactorWordLen=16  derotateFactorDataTypeStr=Inherit: Same word length as input  derotateFactorLastDataTypeStr=Inherit: Same word length as input  denormFactorWordLen=16  denormFactorDataTypeStr=Inherit: Same word length as input  denormFactorLastDataTypeStr=Inherit: Same word length as input  prodOutWordLen=32  prodOutOverflowMode=Wrap  prodOutRoundingMode=Floor  prodOutOvFlMode=off  prodOutOvFlModeLastStrValue=off  sumWordLen=32
  Shift Arithmetic1 : ArithShift  BinPtShiftNumber=-3  BitShiftDirection=Right
  Shift Arithmetic2 : ArithShift  BinPtShiftNumber=3  BitShiftDirection=Right
  Shift Arithmetic3 : ArithShift  BinPtShiftNumber=3  BitShiftDirection=Right
  Sum of Elements : Sum  Inputs=+  OutDataTypeStr=fixdt(0,3,0)
  Symbol Accum1 : Subsystem
  Unit Delay Enabled1 : simulink_need_slupdate/Unit Delay Enabled  Commented=on  vinit=0.0  tsamp=-1
  BER : Outport  InitialOutput=0  VectorParamsAs1DForOutWhenUnconnected=off
  wires:
  " Integrate and Dump"/2(sumOut) -> Delay11/1
  " Integrate and Dump"/1(validOut) -> Delay6/1
  Delay11/1 -> Data Type Conversion2/1
  pilotValid/1 -> Delay10/1
  Data Type Conversion2/1 -> Shift Arithmetic3/1
  Code/1 -> Delay12/1
  Delay12/1 -> Product2/2
  pilotChips/1 -> Delay16/1
  Product2/1 -> Delay9/1
  Shift Arithmetic1/1 -> Product2/1
  Conjugate/1 -> Shift Arithmetic1/1
  chipValid/1 -> Delay15/1
  chips/1 -> Delay13/1
  Delay15/1 -> Symbol Accum1/1(SwCtrl)
  Delay16/1 -> Conjugate/1
  Rectangular QAM Demodulator Baseband1/1 -> Delay17/1
  Rectangular QAM Demodulator Baseband2/1 -> Delay18/1
  Bitwise Operator/1 -> Sum of Elements/1
  Delay17/1 -> Bitwise Operator/2
  Delay18/1 -> Bitwise Operator/1
  Delay10/1 -> " Integrate and Dump1"/1(dValid), " Integrate and Dump"/1(dValid)
  Delay9/1 -> " Integrate and Dump"/2(symbolIn)
  Data Type Conversion3/1 -> Shift Arithmetic2/1
  Delay20/1 -> Data Type Conversion3/1
  " Integrate and Dump1"/2(sumOut) -> Delay20/1
  " Integrate and Dump1"/1(validOut) -> Delay21/1
  Delay13/1 -> " Integrate and Dump1"/2(symbolIn)
  Sum of Elements/1 -> Delay14/1
  Delay14/1 -> Symbol Accum1/2(In)
  BER Avg/1(avgVecOut) -> BER/1
  Symbol Accum1/1(Out) -> BER Avg/1(codeVec)
  Symbol Accum1/2(ValidOut) -> BER Avg/2(enable)
  Shift Arithmetic2/1 -> Delay19/1
  Shift Arithmetic3/1 -> Delay22/1
  Delay19/1 -> Rectangular QAM Demodulator Baseband2/1
  Delay22/1 -> Rectangular QAM Demodulator Baseband1/1

== system benchlink/HDL_64QAM/HDLRxIPCore/QAM Rx HDL/MF Filtering and Despreading/Channel Estimation ==
  isValidSym : Inport
  isAccessSym : Inport  Port=2
  AccessSymVec : Inport  Port=3
  ChipVec : Inport  Port=4
  Accum Scale : Gain  Gain=1/N/rms(AccessSym)^2  OutDataTypeStr=fixdt(1,32,28)  SaturateOnIntegerOverflow=on
  Add2 : Sum  OutDataTypeStr=fixdt(1,32,21)  SaturateOnIntegerOverflow=on
  Constant1 : Constant  Value=complex(0,0)  OutDataTypeStr=fixdt(1,32,21)  SampleTime=1/qam_params.chipRate
  Delay1 : Delay  DelayLength=N  InitialCondition=0
  Delay6 : Delay  DelayLength=1  InitialCondition=0
  Enabled Wire : Subsystem  TreatAsAtomicUnit=on
  Enabled Wire1 : Subsystem  TreatAsAtomicUnit=on
  Falling Edge Detector : Subsystem
  Product of Elements : Product  SaturateOnIntegerOverflow=on
  SEL2 : MultiPortSwitch  DataPortOrder=Zero-based contiguous  Inputs=2  DiagnosticForDefault=None  zeroidx=on  OutDataTypeStr=fixdt(1,32,21)  InputSameDT=off
  Signal Specification : SignalSpecification  Dimensions=1
  Unit Delay1 : UnitDelay  InitialCondition=0+0j  SampleTime=-1  HasFrameUpgradeWarning=on
  ChannelCoeff : Outport  VectorParamsAs1DForOutWhenUnconnected=off
  wires:
  Falling Edge Detector/1(Out1) -> Enabled Wire/Enable
  Unit Delay1/1 -> SEL2/3, Accum Scale/1
  SEL2/1 -> Add2/1
  Accum Scale/1 -> Enabled Wire/1(In1)
  Add2/1 -> Unit Delay1/1
  Product of Elements/1 -> Add2/2
  Constant1/1 -> SEL2/2
  Signal Specification/1 -> ChannelCoeff/1
  AccessSymVec/1 -> Product of Elements/1
  ChipVec/1 -> Product of Elements/2
  Enabled Wire/1(Out1) -> Enabled Wire1/1(In1)
  Enabled Wire1/1(Out1) -> Delay6/1
  Delay1/1 -> Enabled Wire1/Enable
  isValidSym/1 -> Delay1/1
  isAccessSym/1 -> Falling Edge Detector/1(In1), SEL2/1
  Delay6/1 -> Signal Specification/1

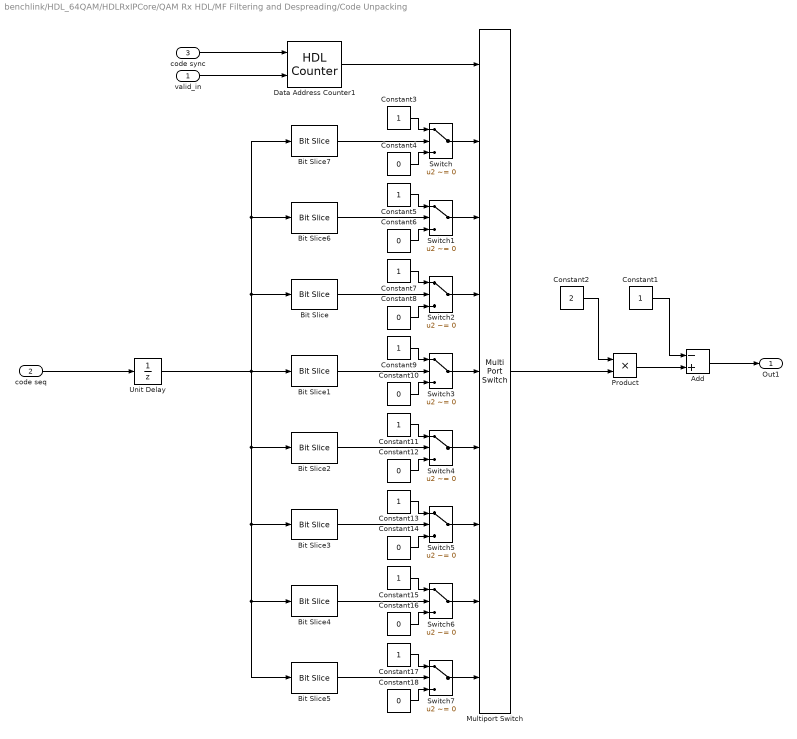
== system benchlink/HDL_64QAM/HDLRxIPCore/QAM Rx HDL/MF Filtering and Despreading/Code Unpacking ==
  valid_in : Inport
  code seq : Inport  Port=2
  code sync : Inport  Port=3
  Add : Sum  Inputs=-+  OutDataTypeStr=fixdt(1,16,14)  SaturateOnIntegerOverflow=on
  Bit Slice : hdlsllib/Logic and Bit Operations/Bit Slice  lidx=5  ridx=5
  Bit Slice1 : hdlsllib/Logic and Bit Operations/Bit Slice  lidx=4  ridx=4
  Bit Slice2 : hdlsllib/Logic and Bit Operations/Bit Slice  lidx=3  ridx=3
  Bit Slice3 : hdlsllib/Logic and Bit Operations/Bit Slice  lidx=2  ridx=2
  Bit Slice4 : hdlsllib/Logic and Bit Operations/Bit Slice  lidx=1  ridx=1
  Bit Slice5 : hdlsllib/Logic and Bit Operations/Bit Slice  lidx=0  ridx=0
  Bit Slice6 : hdlsllib/Logic and Bit Operations/Bit Slice  lidx=6  ridx=6
  Bit Slice7 : hdlsllib/Logic and Bit Operations/Bit Slice  lidx=7  ridx=7
  Constant1 : Constant  OutDataTypeStr=boolean  SampleTime=-1
  Constant{4,6,8,10,12,14,16,18} (8 alike) : Constant  Value=0  OutDataTypeStr=boolean  SampleTime=1/(qam_params.chipRate)
  Constant{3,5,7,9,11,13,15,17} (8 alike) : Constant  OutDataTypeStr=boolean  SampleTime=1/(qam_params.chipRate)
  Constant2 : Constant  Value=2  OutDataTypeStr=fixdt(1,16,0)  SampleTime=-1
  Data Address Counter1 : hdlsllib/Sources/HDL Counter  CountType=Count limited  CountInit=1  CountStep=1  CountMax=qam_params.spreadingFactor  CountFromType=Initial value  CountFrom=1  CountResetPort=on  CountLoadPort=off  CountEnbPort=on  CountDirPort=off  CountHitOutputPort=off  CountDataType=Unsigned  CountWordLen=16  CountFracLen=0  CountSampTime=-1
  Multiport Switch : MultiPortSwitch  Inputs=8  InputSameDT=off
  Product : Product  SaturateOnIntegerOverflow=on
  Switch{,1..7} (8 alike) : Switch  Criteria=u2 ~= 0  InputSameDT=off
  Unit Delay : UnitDelay  InitialCondition=int16(165)  SampleTime=-1  HasFrameUpgradeWarning=on
  Out1 : Outport  VectorParamsAs1DForOutWhenUnconnected=off
  wires:
  Product/1 -> Add/2
  Constant2/1 -> Product/1
  Constant1/1 -> Add/1
  Data Address Counter1/1 -> Multiport Switch/1
  valid_in/1 -> Data Address Counter1/2
  code sync/1 -> Data Address Counter1/1
  Constant16/1 -> Switch6/3
  Bit Slice3/1 -> Switch5/2
  Constant17/1 -> Switch7/1
  Switch7/1 -> Multiport Switch/9
  Constant14/1 -> Switch5/3
  Switch5/1 -> Multiport Switch/7
  Bit Slice1/1 -> Switch3/2
  Bit Slice7/1 -> Switch/2
  Constant13/1 -> Switch5/1
  Switch4/1 -> Multiport Switch/6
  Switch3/1 -> Multiport Switch/5
  Bit Slice4/1 -> Switch6/2
  Constant11/1 -> Switch4/1
  Switch/1 -> Multiport Switch/2
  Bit Slice/1 -> Switch2/2
  Switch6/1 -> Multiport Switch/8
  Switch2/1 -> Multiport Switch/4
  Constant10/1 -> Switch3/3
  Bit Slice5/1 -> Switch7/2
  Bit Slice2/1 -> Switch4/2
  Constant18/1 -> Switch7/3
  Constant12/1 -> Switch4/3
  Switch1/1 -> Multiport Switch/3
  Constant6/1 -> Switch1/3
  Constant7/1 -> Switch2/1
  Constant15/1 -> Switch6/1
  Constant9/1 -> Switch3/1
  Unit Delay/1 -> Bit Slice2/1, Bit Slice3/1, Bit Slice4/1, Bit Slice5/1, Bit Slice6/1, Bit Slice7/1, Bit Slice/1, Bit Slice1/1
  Bit Slice6/1 -> Switch1/2
  Constant3/1 -> Switch/1
  Constant5/1 -> Switch1/1
  Constant4/1 -> Switch/3
  Constant8/1 -> Switch2/3
  Multiport Switch/1 -> Product/2
  code seq/1 -> Unit Delay/1
  Add/1 -> Out1/1

== system benchlink/HDL_64QAM/HDLRxIPCore/QAM Rx HDL/MF Filtering and Despreading/Desired Symbol Source ==
  Enable : Inport
  Code : Inport  Port=2
  Delay{1..3,5} (4 alike) : Delay  DelayLength=1  InitialCondition=0
  HDL Counter1 : hdlsllib/Sources/HDL Counter  CountType=Count limited  CountInit=0  CountStep=1  CountMax=qam_params.spreadingFactor-1  CountFromType=Initial value  CountFrom=0  CountResetPort=on  CountLoadPort=off  CountEnbPort=on  CountDirPort=off  CountHitOutputPort=off  CountDataType=Unsigned  CountWordLen=16  CountFracLen=0  CountSampTime=-1
  HDL Counter2 : hdlsllib/Sources/HDL Counter  CountType=Count limited  CountInit=0  CountStep=1  CountMax=N-1  CountFromType=Initial value  CountFrom=0  CountResetPort=on  CountLoadPort=off  CountEnbPort=on  CountDirPort=off  CountHitOutputPort=off  CountDataType=Unsigned  CountWordLen=16  CountFracLen=0  CountSampTime=-1
  Product1 : Product  OutDataTypeStr=fixdt(1,16,15)  RndMeth=Zero
  Product2 : Product  OutDataTypeStr=fixdt(1,16,15)  RndMeth=Zero
  Rising Edge Detector : Subsystem
  To Workspace4 : ToWorkspace  VariableName=yout407  SampleTime=-1
      settings: Save2DSignal=2-D array (concatenate along first dimension)
  data lookup : LookupNDDirect  NumberOfTableDimensions=1  Table=conj(AccessSym)  DiagnosticForOutOfRangeInput=Error  TableDataTypeStr=fixdt(1,16,15)
  data lookup1 : LookupNDDirect  NumberOfTableDimensions=1  Table=qam_params.codeSequence.'  DiagnosticForOutOfRangeInput=Error  TableDataTypeStr=fixdt(1,16,14)
  Output : Outport  VectorParamsAs1DForOutWhenUnconnected=off
  wires:
  HDL Counter2/1 -> data lookup/1
  data lookup/1 -> Product1/1
  Delay5/1 -> Output/1
  Enable/1 -> Rising Edge Detector/1(In1), Delay1/1
  data lookup1/1 -> Product1/2
  Product2/1 -> Delay5/1
  Product1/1 -> Delay2/1
  HDL Counter1/1 -> data lookup1/1
  Delay2/1 -> Product2/1
  Code/1 -> Delay3/1
  Delay3/1 -> Product2/2, To Workspace4/1
  Rising Edge Detector/1(Out1) -> HDL Counter2/1, HDL Counter1/1
  Delay1/1 -> HDL Counter2/2, HDL Counter1/2

== system benchlink/HDL_64QAM/HDLRxIPCore/QAM Rx HDL/MF Filtering and Despreading/Normalized MF FIlter ==
  ChannelCoeff : Inport
  CodeVec : Inport  Port=2
  EQEnable : Inport  Port=3
  Complex to Magnitude-Angle HDL Optimized : dsphdlmathfun2/Complex to Magnitude-Angle  NumIterationsSource=Property  NumIterations=15  OutputFormat=Magnitude and angle  AngleFormat=Normalized  ScaleOutput=on  ScalingMethod=Shift-Add  SimulateUsing=Code generation
  Conjugate : Math  Operator=conj  SignedPower=on  RndMeth=Zero
  Constant : Constant  OutDataTypeStr=boolean  SampleTime=1/(qam_params.chipRate)
  Constant2 : Constant  Value=complex(sqrt(8*0.875),0)  VectorParams1D=off  OutDataTypeStr=fixdt(1,16,8)  SampleTime=1/(qam_params.chipRate)
  Cosine HDL Optimized : hdlsllib/Lookup Tables/Cosine HDL Optimized  OutputFormula=exp(j*2*pi*u)  NumDataPoints=256  TableDataTypeStr=fixdt(0,31,20)  SimulateLUTROMDelay=off
  Data Type Conversion : DataTypeConversion  OutDataTypeStr=fixdt(1,16,12)  RndMeth=Floor
  Delay{1..7,13,17} (9 alike) : Delay  DelayLength=1  InitialCondition=0
  Delay16 : Delay  DelayLength=23  InitialCondition=0
  Gain1 : Gain  Gain=1/qam_params.spreadingFactor  OutDataTypeStr=fixdt(1,16,14)  SaturateOnIntegerOverflow=on
  Gain3 : Gain  Gain=1/2  OutDataTypeStr=fixdt(1,16,15)  SaturateOnIntegerOverflow=on
  Product : Product  OutDataTypeStr=fixdt(1,32,18)  SaturateOnIntegerOverflow=on
  Product1 : Product  OutDataTypeStr=fixdt(1,16,8)  SaturateOnIntegerOverflow=on
  Reciprocal : Product  Inputs=/  OutDataTypeStr=fixdt(1,12,4)  RndMeth=Zero  SaturateOnIntegerOverflow=on
  Signal Specification : SignalSpecification  Dimensions=1
  Switch9 : Switch  Criteria=u2 ~= 0  SaturateOnIntegerOverflow=off  InputSameDT=off
  Terminator : Terminator
  wMF_N : Outport  VectorParamsAs1DForOutWhenUnconnected=off
  wires:
  Delay16/1 -> Product/2
  CodeVec/1 -> Delay13/1
  Gain1/1 -> Delay16/1
  Delay4/1 -> Switch9/1
  Product/1 -> Delay17/1
  Delay17/1 -> wMF_N/1
  ChannelCoeff/1 -> Delay1/1
  Delay13/1 -> Gain1/1
  Product1/1 -> Delay4/1
  Constant/1 -> Complex to Magnitude-Angle HDL Optimized/2
  Data Type Conversion/1 -> Delay2/1
  Signal Specification/1 -> Cosine HDL Optimized/1
  Complex to Magnitude-Angle HDL Optimized/1 -> Delay3/1
  Complex to Magnitude-Angle HDL Optimized/2 -> Delay5/1
  Conjugate/1 -> Data Type Conversion/1
  Cosine HDL Optimized/1 -> Delay7/1
  Gain3/1 -> Signal Specification/1
  Reciprocal/1 -> Delay6/1
  Complex to Magnitude-Angle HDL Optimized/3 -> Terminator/1
  Delay2/1 -> Complex to Magnitude-Angle HDL Optimized/1
  Delay3/1 -> Reciprocal/1
  Delay5/1 -> Gain3/1
  Delay6/1 -> Product1/1
  Delay7/1 -> Product1/2
  Delay1/1 -> Conjugate/1
  EQEnable/1 -> Switch9/2
  Constant2/1 -> Switch9/3
  Switch9/1 -> Product/1

== system benchlink/HDL_64QAM/HDLRxIPCore/QAM Rx HDL/MF Filtering and Despreading/Rising Edge Detector ==
  In1 : Inport
  Compare To Constant7 : simulink/Logic and Bit Operations/Compare To Constant  relop===  const=1  OutDataTypeStr=boolean
  Data Type Conversion : DataTypeConversion  OutDataTypeStr=fixdt(1,2,0)  SaturateOnIntegerOverflow=off  RndMeth=Floor
  Data Type Conversion1 : DataTypeConversion  OutDataTypeStr=fixdt(1,2,0)  SaturateOnIntegerOverflow=off  RndMeth=Floor
  Data Type Conversion2 : DataTypeConversion  OutDataTypeStr=fixdt(1,2,0)  SaturateOnIntegerOverflow=off  RndMeth=Floor
  Delay1 : Delay  DelayLength=1  InitialCondition=0
  Subtract1 : Sum  Inputs=-+
  code sync : Outport  VectorParamsAs1DForOutWhenUnconnected=off
  wires:
  In1/1 -> Data Type Conversion1/1, Delay1/1
  Delay1/1 -> Data Type Conversion/1
  Subtract1/1 -> Data Type Conversion2/1
  Data Type Conversion/1 -> Subtract1/1
  Data Type Conversion1/1 -> Subtract1/2
  Data Type Conversion2/1 -> Compare To Constant7/1
  Compare To Constant7/1 -> code sync/1
